simulink model "axi_qpsk_rx_tsync"  (R2017b)
settings: Solver=VariableStepAuto  StartTime=0.0  StopTime=10.0  RelTol=1e-3
PreLoadFcn:
  | fs_in = 25.6e6;
  | 
  | design_filters_rx;      % run script to generate filter designs.
  | 
  | Rb = 1000;   % 1kbit / s
  | 
  | Rsym = Rb/2;   % 2 bits per symbol
  | 
  | Rsymbol = Rb/2;
  | 
  | OSR = 32;
  | 
  | f_error = 120;
  | 
  | fc = 100e3;
undefined symbols (not defined in the file or in its folder): AXI4, Lite
libraries: xbsIndex_r4 x239
(part 1 of 2)
settings Model: Creator=jgoldsmi  LastModifiedBy=jgoldsmi

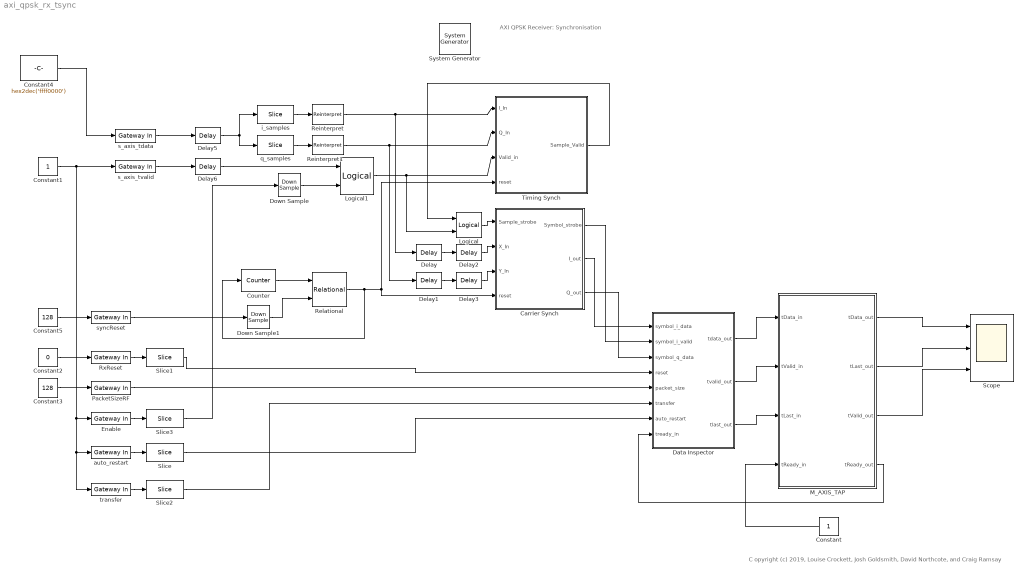
== system axi_qpsk_rx_tsync ==
  note: C opyright (c) 2019, Louise Crockett, Josh Goldsmith, David Northcote, and Craig Ramsay
  note: AXI QPSK Receiver:
      | Synchronisation
  " System Generator" : xbsIndex_r4/ System Generator  Tag=genX  xilinxfamily=zynquplusRFSOC  part=xczu28dr  speed=-2-e  package=ffvg1517  synthesis_tool=Vivado  clock_wrapper=Clock Enables  directory=Y:/git/craig_repo/rfsoc_qpsk_demo/boards/ip/sysgen/iprepo/zcu111/rx_stages/rx_tsync  proj_type=Vivado  Synth_file=Vivado Synthesis Defaults  Impl_file=Vivado Implementation Defaults  testbench=off  simulink_period=1/fs_in  sysclk_period=(1/fs_in)/1e-9  dcm_input_clock_period=10  incr_netlist=off  trim_vbits=Everywhere in SubSystem  dbl_ovrd=According to Block Masks  core_generation=According to Block Masks  run_coregen=off  deprecated_control=off  eval_field=0  block_type=sysgen
  Carrier Synch : Subsystem  mask(Symbol Timing Synchroniser){Rsymbol=Rsymbol}
      mask prompts: Rsymbol "Symbol rate (Hz)"
      mask init:
      | d = 0.707;                  % damping ratio 
      | 
      | % *** CARRIER synch loop *** (note this operates at symbol rate)
      | 
      | T = 1/Rsymbol;               % sample period
      | Kp = 1;                      % phase detector S-curve is linear
      | Bn = 0.04*Rsymbol;           % bandwidth in Hz
      | Ko = 1;                      % gain of NCO 
      | 
      | % calculate the loop filter coefficients for the carrier synch loop
      | K1 = (4*d*Bn*T)/(Ko*Kp*(d+1/(4*d)));
      | K2 = (4*(Bn*T)^2)/(Ko*Kp*(d+1/4*d)^2);
  Constant : Constant  OutDataTypeStr=boolean  SampleTime=1/fs_in
  Constant1 : Constant  OutDataTypeStr=boolean  SampleTime=-1
  Constant2 : Constant  Value=0  OutDataTypeStr=boolean  SampleTime=-1
  Constant3 : Constant  Value=128  OutDataTypeStr=uint32  SampleTime=-1
  Constant4 : Constant  Value=hex2dec('ffff0000')  OutDataTypeStr=uint32  SampleTime=1/fs_in
  Constant5 : Constant  Value=128  OutDataTypeStr=uint32  SampleTime=-1
  Counter : xbsIndex_r4/Counter  cnt_type=Free Running  cnt_to=Inf  operation=Up  start_count=1  cnt_by_val=1  arith_type=Unsigned  n_bits=32  bin_pt=0  load_pin=off  rst=on  en=off  explicit_period=on  period=1/16e3  use_behavioral_HDL=off  implementation=Fabric  dbl_ovrd=off  block_type=counter
  Data Inspector : Subsystem
  Delay : xbsIndex_r4/Delay  rst=off  infoeditControl=Selection of Reset will increase slice count due to use of real FFs and instead of SRLs  en=off  latency=OSR/2  reg_retiming=off  dbl_ovrd=off  block_type=delay
  Delay1 : xbsIndex_r4/Delay  rst=off  infoeditControl=Selection of Reset will increase slice count due to use of real FFs and instead of SRLs  en=off  latency=OSR/2  reg_retiming=off  dbl_ovrd=off  block_type=delay
  Delay{2..3,5..6} (4 alike) : xbsIndex_r4/Delay  rst=off  infoeditControl=Selection of Reset will increase slice count due to use of real FFs and instead of SRLs  en=off  latency=1  reg_retiming=off  dbl_ovrd=off  block_type=delay
  Down Sample : xbsIndex_r4/Down Sample  sample_ratio=1600  sample_phase="Last Value of Frame  (most efficient)"  en=off  rst=off  latency=1  dbl_ovrd=off  block_type=dsamp
  Down Sample1 : xbsIndex_r4/Down Sample  sample_ratio=1600  sample_phase="Last Value of Frame  (most efficient)"  en=off  rst=off  latency=1  dbl_ovrd=off  block_type=dsamp
  Enable : xbsIndex_r4/Gateway In  gui_display_data_type=Fixed-point  arith_type=Unsigned  n_bits=32  bin_pt=0  preci_type=Single  exp_width=8  frac_width=24  rows=1  columns=1  quantization="Round  (unbiased: +/- Inf)"  overflow=Saturate  period=1/fs_in  UseAsADC=off  ADCChannel='1'  interface=AXI4-Lite  automatic_assignment=off  address_offset=8  intf_name=''  intf_description=''  default_value=0  timing_constraint=None  locs_specified=off  LOCs={}  io_standard={}  inherit_from_input=off  hdl_port=on  dbl_ovrd=off  block_type=gatewayin
  Logical : xbsIndex_r4/Logical  logical_function=AND  inputs=2  en=off  latency=0  precision=Full  arith_type=Unsigned  n_bits=16  bin_pt=0  align_bp=on  dbl_ovrd=off  block_type=logical
  Logical1 : xbsIndex_r4/Logical  logical_function=AND  inputs=2  en=off  latency=0  precision=Full  arith_type=Unsigned  n_bits=16  bin_pt=0  align_bp=on  dbl_ovrd=off  block_type=logical
  M_AXIS_TAP : Subsystem
  PacketSizeRF : xbsIndex_r4/Gateway In  gui_display_data_type=Fixed-point  arith_type=Unsigned  n_bits=32  bin_pt=0  preci_type=Single  exp_width=8  frac_width=24  rows=1  columns=1  quantization=Truncate  overflow=Wrap  period=1/fs_in  UseAsADC=off  ADCChannel='1'  interface=AXI4-Lite  automatic_assignment=off  address_offset=4  intf_name=''  intf_description=''  default_value=0  timing_constraint=None  locs_specified=off  LOCs={}  io_standard={}  inherit_from_input=off  hdl_port=on  dbl_ovrd=off  block_type=gatewayin
  Reinterpret : xbsIndex_r4/Reinterpret  force_arith_type=on  arith_type="Signed  (2's comp)"  force_bin_pt=on  bin_pt=14  block_type=reinterpret
  Reinterpret1 : xbsIndex_r4/Reinterpret  force_arith_type=on  arith_type="Signed  (2's comp)"  force_bin_pt=on  bin_pt=14  block_type=reinterpret
  Relational : xbsIndex_r4/Relational  mode=a=b  op_type=Bool  en=off  latency=0  dbl_ovrd=off  block_type=relational
  RxReset : xbsIndex_r4/Gateway In  gui_display_data_type=Fixed-point  arith_type=Unsigned  n_bits=32  bin_pt=0  preci_type=Single  exp_width=8  frac_width=24  rows=1  columns=1  quantization="Round  (unbiased: +/- Inf)"  overflow=Saturate  period=1/fs_in  UseAsADC=off  ADCChannel='1'  interface=AXI4-Lite  automatic_assignment=off  address_offset=0  intf_name=''  intf_description=''  default_value=0  timing_constraint=None  locs_specified=off  LOCs={}  io_standard={}  inherit_from_input=off  hdl_port=on  dbl_ovrd=off  block_type=gatewayin
  Scope : Scope  NumInputPorts=3
  Slice{,1..3} (4 alike) : xbsIndex_r4/Slice  nbits=1  boolean_output=on  mode=Two Bit Locations  bit1=0  base1=LSB of Input  bit0=0  base0=LSB of Input  dbl_ovrd=off  block_type=slice
  Timing Synch : Subsystem  mask(Symbol Timing Synchroniser){Rsymbol=Rsymbol}
      mask prompts: Rsymbol "Symbol rate (Hz)"
      mask init:
      | % *** SYMBOL TIMING synch loop ***
      | 
      | d = 0.707;                  % damping ratio 
      | Ts = 1/Rsymbol;             % symbol period
      | Ks = 3.24;                  % phase detector coefficient
      | BnS = 0.08*Rsymbol;         % bandwidth in Hz
      | Kn   = 1;                   % gain of numerically controlled clock
      | 
      | % calculate loop filter coefficients
      | Ka = (4*d*BnS*Ts)/(Kn*Ks*(d+1/(4*d)));
      | Kb = (4*(BnS*Ts)^2)/(Kn*Ks*(d+1/4*d)^2);
  auto_restart : xbsIndex_r4/Gateway In  gui_display_data_type=Fixed-point  arith_type=Unsigned  n_bits=32  bin_pt=0  preci_type=Single  exp_width=8  frac_width=24  rows=1  columns=1  quantization="Round  (unbiased: +/- Inf)"  overflow=Saturate  period=1/fs_in  UseAsADC=off  ADCChannel='1'  interface=AXI4-Lite  automatic_assignment=off  address_offset=12  intf_name=''  intf_description=''  default_value=0  timing_constraint=None  locs_specified=off  LOCs={}  io_standard={}  inherit_from_input=off  hdl_port=on  dbl_ovrd=off  block_type=gatewayin
  i_samples : xbsIndex_r4/Slice  nbits=16  boolean_output=off  mode=Upper Bit Location + Width  bit1=0  base1=MSB of Input  bit0=0  base0=LSB of Input  dbl_ovrd=off  block_type=slice
  q_samples : xbsIndex_r4/Slice  nbits=16  boolean_output=off  mode=Lower Bit Location + Width  bit1=0  base1=MSB of Input  bit0=0  base0=LSB of Input  dbl_ovrd=off  block_type=slice
  s_axis_tdata : xbsIndex_r4/Gateway In  gui_display_data_type=Fixed-point  arith_type=Unsigned  n_bits=32  bin_pt=0  preci_type=Single  exp_width=8  frac_width=24  rows=1  columns=1  quantization="Round  (unbiased: +/- Inf)"  overflow=Saturate  period=1/16e3  UseAsADC=off  ADCChannel='1'  interface=None  automatic_assignment=on  address_offset=hex2dec('00')  intf_name=''  intf_description=''  default_value=0  timing_constraint=None  locs_specified=off  LOCs={}  io_standard={}  inherit_from_input=off  hdl_port=on  dbl_ovrd=off  block_type=gatewayin
  s_axis_tvalid : xbsIndex_r4/Gateway In  gui_display_data_type=Boolean  arith_type=Boolean  n_bits=32  bin_pt=0  preci_type=Single  exp_width=8  frac_width=24  rows=1  columns=1  quantization="Round  (unbiased: +/- Inf)"  overflow=Saturate  period=1/16e3  UseAsADC=off  ADCChannel='1'  interface=None  automatic_assignment=on  address_offset=hex2dec('00')  intf_name=''  intf_description=''  default_value=0  timing_constraint=None  locs_specified=off  LOCs={}  io_standard={}  inherit_from_input=off  hdl_port=on  dbl_ovrd=off  block_type=gatewayin
  syncReset : xbsIndex_r4/Gateway In  gui_display_data_type=Fixed-point  arith_type=Unsigned  n_bits=32  bin_pt=0  preci_type=Single  exp_width=8  frac_width=24  rows=1  columns=1  quantization=Truncate  overflow=Wrap  period=1/fs_in  UseAsADC=off  ADCChannel='1'  interface=AXI4-Lite  automatic_assignment=off  address_offset=20  intf_name=''  intf_description=''  default_value=0  timing_constraint=None  locs_specified=off  LOCs={}  io_standard={}  inherit_from_input=off  hdl_port=on  dbl_ovrd=off  block_type=gatewayin
  transfer : xbsIndex_r4/Gateway In  gui_display_data_type=Fixed-point  arith_type=Unsigned  n_bits=32  bin_pt=0  preci_type=Single  exp_width=8  frac_width=24  rows=1  columns=1  quantization="Round  (unbiased: +/- Inf)"  overflow=Saturate  period=1/fs_in  UseAsADC=off  ADCChannel='1'  interface=AXI4-Lite  automatic_assignment=off  address_offset=16  intf_name=''  intf_description=''  default_value=0  timing_constraint=None  locs_specified=off  LOCs={}  io_standard={}  inherit_from_input=off  hdl_port=on  dbl_ovrd=off  block_type=gatewayin
  wires:
  RxReset/1 -> Slice1/1
  Enable/1 -> Slice3/1
  auto_restart/1 -> Slice/1
  transfer/1 -> Slice2/1
  Constant2/1 -> RxReset/1
  Constant1/1 -> transfer/1, auto_restart/1, Enable/1, s_axis_tvalid/1
  Constant3/1 -> PacketSizeRF/1
  M_AXIS_TAP/3(tValid_out) -> Scope/3
  Constant/1 -> M_AXIS_TAP/4(tReady_in)
  Data Inspector/3(tlast_out) -> M_AXIS_TAP/3(tLast_in)
  M_AXIS_TAP/1(tData_out) -> Scope/1
  M_AXIS_TAP/2(tLast_out) -> Scope/2
  M_AXIS_TAP/4(tReady_out) -> Data Inspector/8(tready_in)
  Data Inspector/2(tvalid_out) -> M_AXIS_TAP/2(tValid_in)
  Data Inspector/1(tdata_out) -> M_AXIS_TAP/1(tData_in)
  Delay/1 -> Delay2/1
  Delay3/1 -> Carrier Synch/3(Y_In)
  Delay2/1 -> Carrier Synch/2(X_In)
  Timing Synch/1(Sample_Valid) -> Logical/1
  Logical/1 -> Carrier Synch/1(Sample_strobe)
  Delay1/1 -> Delay3/1
  i_samples/1 -> Reinterpret/1
  q_samples/1 -> Reinterpret1/1
  Slice1/1 -> Data Inspector/4(reset)
  PacketSizeRF/1 -> Data Inspector/5(packet_size)
  Logical1/1 -> Logical/2, Timing Synch/3(Valid_in)
  Slice3/1 -> Down Sample/1
  Slice/1 -> Data Inspector/7(auto_restart)
  Slice2/1 -> Data Inspector/6(transfer)
  Carrier Synch/1(Symbol_strobe) -> Data Inspector/2(symbol_i_valid)
  Down Sample/1 -> Logical1/2
  Constant4/1 -> s_axis_tdata/1
  Carrier Synch/2(I_out) -> Data Inspector/1(symbol_i_data)
  Carrier Synch/3(Q_out) -> Data Inspector/3(symbol_q_data)
  Constant5/1 -> syncReset/1
  s_axis_tdata/1 -> Delay5/1
  s_axis_tvalid/1 -> Delay6/1
  Reinterpret/1 -> Delay/1, Timing Synch/1(I_In)
  Reinterpret1/1 -> Delay1/1, Timing Synch/2(Q_In)
  Delay6/1 -> Logical1/1
  Delay5/1 -> q_samples/1, i_samples/1
  syncReset/1 -> Down Sample1/1
  Relational/1 -> Counter/1, Carrier Synch/4(reset), Timing Synch/4(reset)
  Counter/1 -> Relational/1
  Down Sample1/1 -> Relational/2

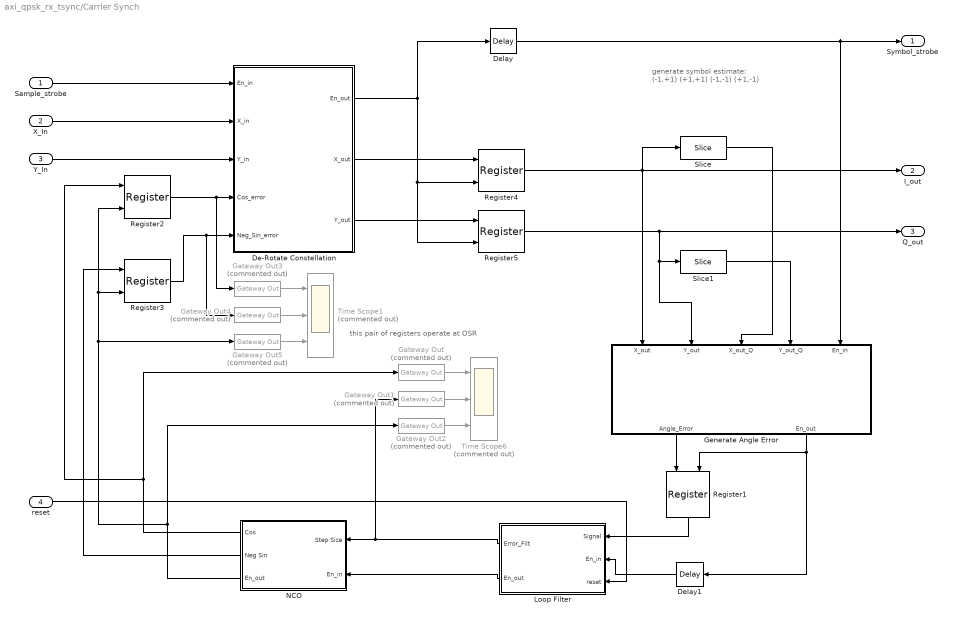
== system axi_qpsk_rx_tsync/Carrier Synch ==
  note: this pair of registers operate at OSR
  note: generate symbol estimate:
      |
      |           (-1,+1)                 (+1,+1)
      |
      |
      |           (-1,-1)                  (+1,-1)
  Sample_strobe : Inport
  X_In : Inport  Port=2
  Y_In : Inport  Port=3
  reset : Inport  Port=4
  De-Rotate Constellation : Subsystem
  Delay : xbsIndex_r4/Delay  rst=off  infoeditControl=Selection of Reset will increase slice count due to use of real FFs and instead of SRLs  en=off  latency=1  reg_retiming=off  dbl_ovrd=off  block_type=delay
  Delay1 : xbsIndex_r4/Delay  rst=off  infoeditControl=Selection of Reset will increase slice count due to use of real FFs and instead of SRLs  en=off  latency=1  reg_retiming=off  dbl_ovrd=off  block_type=delay
  Gateway Out{,1..5} (6 alike) : xbsIndex_r4/Gateway Out  Commented=on  inherit_from_input=off  hdl_port=on  rows=1  columns=1  UseAsDAC=off  DACChannel='1'  interface=None  automatic_assignment=on  address_offset=hex2dec('00')  intf_name=''  intf_description=''  timing_constraint=None  locs_specified=off  LOCs={}  io_standard={}  block_type=gatewayout
  Generate Angle Error : Subsystem
  Loop Filter : Subsystem  mask(Loop Filter){K1=K1, K2=K2}
      mask prompts: K1 "Proportional gain (K1)"; K2 "Integral gain (K2)"
      mask help:
      | Filters the error signal generated within the Carrier Synchronisation Loop.
      |
      | Key parameters are the gain of the proportional and integral branches.
  NCO : Subsystem  mask(NCO){n=8, b=14}
      mask prompts: n "Number of integer_bits"; b "Number of fractional bits"
      mask help:
      | Numerically Controller Oscillator.
      |
      | Integrates the phase error and generates cosine and negative sign outputs.
      mask init:
      | k_n = ceil(log2((2^n)/(2*pi)))
      mask DialogControl Container3 Prompt: Accumulator
  Register1 : xbsIndex_r4/Register  init=0  rst=off  en=on  dbl_ovrd=off  block_type=register
  Register2 : xbsIndex_r4/Register  init=1  rst=off  en=on  dbl_ovrd=off  block_type=register
  Register3 : xbsIndex_r4/Register  init=0  rst=off  en=on  dbl_ovrd=off  block_type=register
  Register4 : xbsIndex_r4/Register  init=1  rst=off  en=on  dbl_ovrd=off  block_type=register
  Register5 : xbsIndex_r4/Register  init=1  rst=off  en=on  dbl_ovrd=off  block_type=register
  Slice : xbsIndex_r4/Slice  nbits=1  boolean_output=off  mode=Upper Bit Location + Width  bit1=0  base1=MSB of Input  bit0=0  base0=LSB of Input  dbl_ovrd=off  block_type=slice
  Slice1 : xbsIndex_r4/Slice  nbits=1  boolean_output=off  mode=Upper Bit Location + Width  bit1=0  base1=MSB of Input  bit0=0  base0=LSB of Input  dbl_ovrd=off  block_type=slice
  Time Scope1 : Scope  Commented=on  NumInputPorts=3
  Time Scope6 : Scope  Commented=on  NumInputPorts=3
  Symbol_strobe : Outport
  I_out : Outport  Port=2
  Q_out : Outport  Port=3
  wires:
  X_In/1 -> De-Rotate Constellation/2(X_in)
  Y_In/1 -> De-Rotate Constellation/3(Y_in)
  Register4/1 -> Slice/1, I_out/1, Generate Angle Error/1(X_out)
  Register5/1 -> Q_out/1, Generate Angle Error/2(Y_out), Slice1/1
  Slice/1 -> Generate Angle Error/3(X_out_Q)
  Slice1/1 -> Generate Angle Error/4(Y_out_Q)
  Register1/1 -> Loop Filter/1(Signal)
  Loop Filter/2(En_out) -> NCO/2(En_in)
  Loop Filter/1(Error_Filt) -> Gateway Out1/1, NCO/1(Step Size)
  Register2/1 -> Gateway Out3/1, De-Rotate Constellation/4(Cos_error)
  Register3/1 -> Gateway Out4/1, De-Rotate Constellation/5(Neg_Sin_error)
  NCO/1(Cos) -> Gateway Out/1, Register2/1
  NCO/2(Neg Sin) -> Register3/1
  NCO/3(En_out) -> Gateway Out2/1, Gateway Out5/1, Register2/2, Register3/2
  Sample_strobe/1 -> De-Rotate Constellation/1(En_in)
  De-Rotate Constellation/1(En_out) -> Delay/1, Register4/2, Register5/2
  Delay/1 -> Symbol_strobe/1, Generate Angle Error/5(En_in)
  Gateway Out/1 -> Time Scope6/1
  Gateway Out1/1 -> Time Scope6/2
  Gateway Out2/1 -> Time Scope6/3
  Generate Angle Error/1(Angle_Error) -> Register1/1
  Generate Angle Error/2(En_out) -> Delay1/1, Register1/2
  Delay1/1 -> Loop Filter/2(En_in)
  Gateway Out5/1 -> Time Scope1/3
  Gateway Out4/1 -> Time Scope1/2
  Gateway Out3/1 -> Time Scope1/1
  De-Rotate Constellation/2(X_out) -> Register4/1
  De-Rotate Constellation/3(Y_out) -> Register5/1
  reset/1 -> Loop Filter/3(reset)

== system axi_qpsk_rx_tsync/Data Inspector ==
  symbol_i_data : Inport
  symbol_i_valid : Inport  Port=2
  symbol_q_data : Inport  Port=3
  reset : Inport  Port=4
  packet_size : Inport  Port=5
  transfer : Inport  Port=6
  auto_restart : Inport  Port=7
  tready_in : Inport  Port=8
  M_AXIS_SYMBOL_CTRL : Subsystem
  tdata_out : Outport
  tvalid_out : Outport  Port=2
  tlast_out : Outport  Port=3
  wires:
  auto_restart/1 -> M_AXIS_SYMBOL_CTRL/8(auto_restart)
  transfer/1 -> M_AXIS_SYMBOL_CTRL/7(transfer)
  M_AXIS_SYMBOL_CTRL/3(tlast_out) -> tlast_out/1
  M_AXIS_SYMBOL_CTRL/2(tvalid_out) -> tvalid_out/1
  M_AXIS_SYMBOL_CTRL/1(tdata_out) -> tdata_out/1
  tready_in/1 -> M_AXIS_SYMBOL_CTRL/6(tready_in)
  packet_size/1 -> M_AXIS_SYMBOL_CTRL/5(packet_size)
  reset/1 -> M_AXIS_SYMBOL_CTRL/4(reset)
  symbol_q_data/1 -> M_AXIS_SYMBOL_CTRL/3(q_data)
  symbol_i_valid/1 -> M_AXIS_SYMBOL_CTRL/2(tvalid_in)
  symbol_i_data/1 -> M_AXIS_SYMBOL_CTRL/1(i_data)

== system axi_qpsk_rx_tsync/M_AXIS_TAP ==
  tData_in : Inport
  tValid_in : Inport  Port=2
  tLast_in : Inport  Port=3
  tReady_in : Inport  Port=4
  m_axis_tap_tdata : xbsIndex_r4/Gateway Out  inherit_from_input=off  hdl_port=on  rows=1  columns=1  UseAsDAC=off  DACChannel='1'  interface=None  automatic_assignment=on  address_offset=hex2dec('00')  intf_name=''  intf_description=''  timing_constraint=None  locs_specified=off  LOCs={}  io_standard={}  block_type=gatewayout
  m_axis_tap_tlast : xbsIndex_r4/Gateway Out  inherit_from_input=off  hdl_port=on  rows=1  columns=1  UseAsDAC=off  DACChannel='1'  interface=None  automatic_assignment=on  address_offset=hex2dec('00')  intf_name=''  intf_description=''  timing_constraint=None  locs_specified=off  LOCs={}  io_standard={}  block_type=gatewayout
  m_axis_tap_tready : xbsIndex_r4/Gateway In  gui_display_data_type=Boolean  arith_type=Boolean  n_bits=16  bin_pt=14  preci_type=Single  exp_width=8  frac_width=24  rows=1  columns=1  quantization="Round  (unbiased: +/- Inf)"  overflow=Saturate  period=1/fs_in  UseAsADC=off  ADCChannel='1'  interface=None  automatic_assignment=on  address_offset=hex2dec('00')  intf_name=''  intf_description=''  default_value=0  timing_constraint=None  locs_specified=off  LOCs={}  io_standard={}  inherit_from_input=off  hdl_port=on  dbl_ovrd=off  block_type=gatewayin
  m_axis_tap_tvalid : xbsIndex_r4/Gateway Out  inherit_from_input=off  hdl_port=on  rows=1  columns=1  UseAsDAC=off  DACChannel='1'  interface=None  automatic_assignment=on  address_offset=hex2dec('00')  intf_name=''  intf_description=''  timing_constraint=None  locs_specified=off  LOCs={}  io_standard={}  block_type=gatewayout
  tData_out : Outport
  tLast_out : Outport  Port=2
  tValid_out : Outport  Port=3
  tReady_out : Outport  Port=4
  wires:
  m_axis_tap_tready/1 -> tReady_out/1
  tValid_in/1 -> m_axis_tap_tvalid/1
  tLast_in/1 -> m_axis_tap_tlast/1
  tData_in/1 -> m_axis_tap_tdata/1
  m_axis_tap_tdata/1 -> tData_out/1
  m_axis_tap_tvalid/1 -> tValid_out/1
  m_axis_tap_tlast/1 -> tLast_out/1
  tReady_in/1 -> m_axis_tap_tready/1

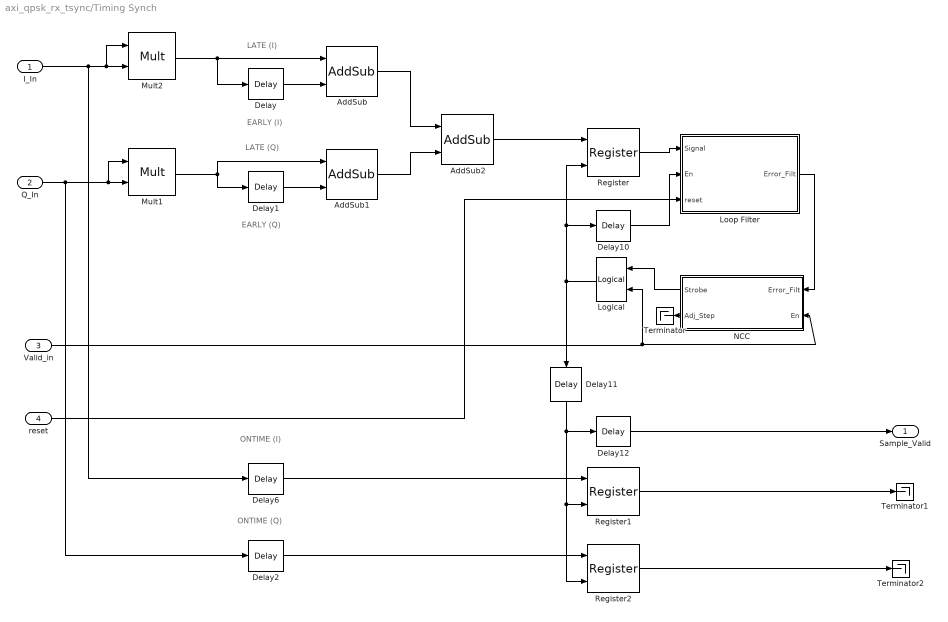
== system axi_qpsk_rx_tsync/Timing Synch ==
  note: LATE (I)
  note: LATE (Q)
  note: EARLY (I)
  note: EARLY (Q)
  note: ONTIME (I)
  note: ONTIME (Q)
  I_In : Inport
  Q_In : Inport  Port=2
  Valid_in : Inport  Port=3
  reset : Inport  Port=4
  AddSub : xbsIndex_r4/AddSub  mode=Subtraction  use_carryin=off  use_carryout=off  en=off  latency=0  precision=Full  arith_type=Unsigned  n_bits=16  bin_pt=14  quantization=Truncate  overflow=Wrap  use_behavioral_HDL=off  hw_selection=Fabric  pipelined=off  dbl_ovrd=off  block_type=addsub
  AddSub1 : xbsIndex_r4/AddSub  mode=Subtraction  use_carryin=off  use_carryout=off  en=off  latency=0  precision=Full  arith_type=Unsigned  n_bits=16  bin_pt=14  quantization=Truncate  overflow=Wrap  use_behavioral_HDL=off  hw_selection=Fabric  pipelined=off  dbl_ovrd=off  block_type=addsub
  AddSub2 : xbsIndex_r4/AddSub  mode=Addition  use_carryin=off  use_carryout=off  en=off  latency=0  precision=Full  arith_type=Unsigned  n_bits=16  bin_pt=14  quantization=Truncate  overflow=Wrap  use_behavioral_HDL=off  hw_selection=Fabric  pipelined=off  dbl_ovrd=off  block_type=addsub
  Delay : xbsIndex_r4/Delay  rst=off  infoeditControl=Selection of Reset will increase slice count due to use of real FFs and instead of SRLs  en=off  latency=OSR  reg_retiming=off  dbl_ovrd=off  block_type=delay
  Delay1 : xbsIndex_r4/Delay  rst=off  infoeditControl=Selection of Reset will increase slice count due to use of real FFs and instead of SRLs  en=off  latency=OSR  reg_retiming=off  dbl_ovrd=off  block_type=delay
  Delay10 : xbsIndex_r4/Delay  rst=off  infoeditControl=Selection of Reset will increase slice count due to use of real FFs and instead of SRLs  en=off  latency=1  reg_retiming=off  dbl_ovrd=off  block_type=delay
  Delay11 : xbsIndex_r4/Delay  rst=off  infoeditControl=Selection of Reset will increase slice count due to use of real FFs and instead of SRLs  en=off  latency=OSR/2  reg_retiming=off  dbl_ovrd=off  block_type=delay
  Delay12 : xbsIndex_r4/Delay  rst=off  infoeditControl=Selection of Reset will increase slice count due to use of real FFs and instead of SRLs  en=off  latency=1  reg_retiming=off  dbl_ovrd=off  block_type=delay
  Delay2 : xbsIndex_r4/Delay  rst=off  infoeditControl=Selection of Reset will increase slice count due to use of real FFs and instead of SRLs  en=off  latency=OSR/2  reg_retiming=off  dbl_ovrd=off  block_type=delay
  Delay6 : xbsIndex_r4/Delay  rst=off  infoeditControl=Selection of Reset will increase slice count due to use of real FFs and instead of SRLs  en=off  latency=OSR/2  reg_retiming=off  dbl_ovrd=off  block_type=delay
  Logical : xbsIndex_r4/Logical  logical_function=AND  inputs=2  en=off  latency=0  precision=Full  arith_type=Unsigned  n_bits=16  bin_pt=0  align_bp=on  dbl_ovrd=off  block_type=logical
  Loop Filter : Subsystem  mask(Loop Filter){Ka=Ka, Kb=Kb}
      mask prompts: Ka "Proportional gain (Ka)"; Kb "Integral gain (Kb)"
      mask help:
      | Filters the error signal generated by the Timing Error Detector.
      |
      | Key parameters are the gain of the proportional and integral branches.
  Mult1 : xbsIndex_r4/Mult  precision=User Defined  arith_type="Signed  (2's comp)"  n_bits=18  bin_pt=14  quantization=Truncate  overflow=Wrap  en=off  latency=0  use_behavioral_HDL=off  opt=Speed  use_embedded=on  optimum_pipeline=off  pipeline=on  dbl_ovrd=off  use_rpm=on  placement_style=Triangular  block_type=mult
  Mult2 : xbsIndex_r4/Mult  precision=User Defined  arith_type="Signed  (2's comp)"  n_bits=18  bin_pt=14  quantization=Truncate  overflow=Wrap  en=off  latency=0  use_behavioral_HDL=off  opt=Speed  use_embedded=on  optimum_pipeline=off  pipeline=on  dbl_ovrd=off  use_rpm=on  placement_style=Triangular  block_type=mult
  NCC : Subsystem  mask(Numerically Controlled Clock (NCC)){OSR=OSR, b=24}
      mask prompts: OSR "Oversampling ratio (nominal samples per symbol)"; b "Fractional bits"
      mask help: Creates strobes at a rate matching the symbol rate of the received data.
      mask init:
      | n = ceil(log2(OSR));
  Register : xbsIndex_r4/Register  init=0  rst=off  en=on  dbl_ovrd=off  block_type=register
  Register1 : xbsIndex_r4/Register  init=0  rst=off  en=on  dbl_ovrd=off  block_type=register
  Register2 : xbsIndex_r4/Register  init=0  rst=off  en=on  dbl_ovrd=off  block_type=register
  Terminator : Terminator
  Terminator1 : Terminator
  Terminator2 : Terminator
  Sample_Valid : Outport
  wires:
  Delay11/1 -> Register2/2, Register1/2, Delay12/1
  Delay/1 -> AddSub/2
  AddSub1/1 -> AddSub2/2
  Mult2/1 -> AddSub/1, Delay/1
  AddSub2/1 -> Register/1
  I_In/1 -> Delay6/1, Mult2/2, Mult2/1
  Q_In/1 -> Delay2/1, Mult1/1, Mult1/2
  Delay10/1 -> Loop Filter/2(En)
  Loop Filter/1(Error_Filt) -> NCC/1(Error_Filt)
  Delay2/1 -> Register2/1
  Delay6/1 -> Register1/1
  Mult1/1 -> Delay1/1, AddSub1/1
  AddSub/1 -> AddSub2/1
  Delay1/1 -> AddSub1/2
  Logical/1 -> Delay11/1, Register/2, Delay10/1
  Register/1 -> Loop Filter/1(Signal)
  Register2/1 -> Terminator2/1
  Delay12/1 -> Sample_Valid/1
  NCC/1(Strobe) -> Logical/1
  Valid_in/1 -> NCC/2(En), Logical/2
  NCC/2(Adj_Step) -> Terminator/1
  Register1/1 -> Terminator1/1
  reset/1 -> Loop Filter/3(reset)

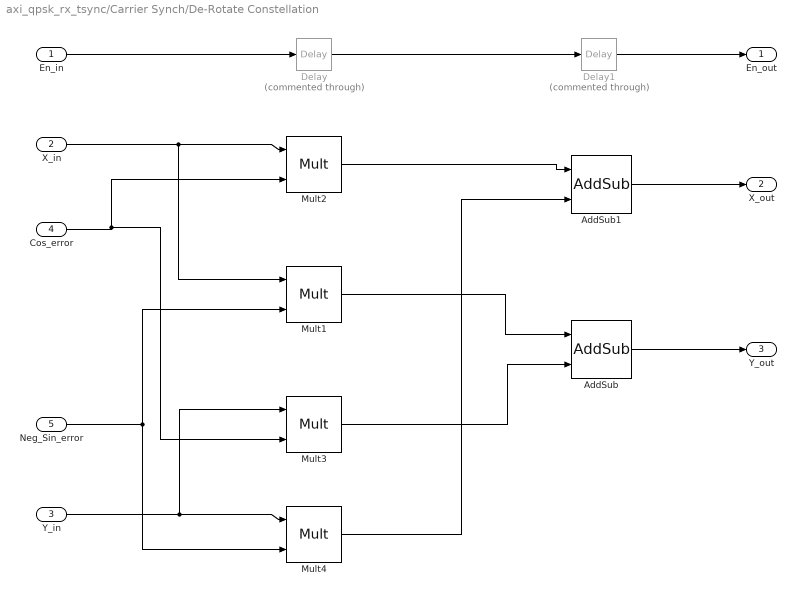
== system axi_qpsk_rx_tsync/Carrier Synch/De-Rotate Constellation ==
  En_in : Inport
  X_in : Inport  Port=2
  Y_in : Inport  Port=3
  Cos_error : Inport  Port=4
  Neg_Sin_error : Inport  Port=5
  AddSub : xbsIndex_r4/AddSub  mode=Addition  use_carryin=off  use_carryout=off  en=off  latency=0  precision=Full  arith_type=Unsigned  n_bits=16  bin_pt=14  quantization=Truncate  overflow=Wrap  use_behavioral_HDL=off  hw_selection=Fabric  pipelined=off  dbl_ovrd=off  block_type=addsub
  AddSub1 : xbsIndex_r4/AddSub  mode=Subtraction  use_carryin=off  use_carryout=off  en=off  latency=0  precision=Full  arith_type=Unsigned  n_bits=16  bin_pt=14  quantization=Truncate  overflow=Wrap  use_behavioral_HDL=off  hw_selection=Fabric  pipelined=off  dbl_ovrd=off  block_type=addsub
  Delay : xbsIndex_r4/Delay  Commented=through  rst=off  infoeditControl=Selection of Reset will increase slice count due to use of real FFs and instead of SRLs  en=off  latency=1  reg_retiming=off  dbl_ovrd=off  block_type=delay
  Delay1 : xbsIndex_r4/Delay  Commented=through  rst=off  infoeditControl=Selection of Reset will increase slice count due to use of real FFs and instead of SRLs  en=off  latency=1  reg_retiming=off  dbl_ovrd=off  block_type=delay
  Mult{1..4} (4 alike) : xbsIndex_r4/Mult  precision=User Defined  arith_type="Signed  (2's comp)"  n_bits=18  bin_pt=14  quantization=Truncate  overflow=Wrap  en=off  latency=0  use_behavioral_HDL=off  opt=Speed  use_embedded=on  optimum_pipeline=off  pipeline=on  dbl_ovrd=off  use_rpm=on  placement_style=Triangular  block_type=mult
  En_out : Outport
  X_out : Outport  Port=2
  Y_out : Outport  Port=3
  wires:
  AddSub1/1 -> X_out/1
  Y_in/1 -> Mult3/1, Mult4/1
  Mult2/1 -> AddSub1/1
  Mult3/1 -> AddSub/2
  Cos_error/1 -> Mult3/2, Mult2/2
  X_in/1 -> Mult1/1, Mult2/1
  Mult1/1 -> AddSub/1
  AddSub/1 -> Y_out/1
  Mult4/1 -> AddSub1/2
  Neg_Sin_error/1 -> Mult4/2, Mult1/2
  En_in/1 -> Delay/1
  Delay/1 -> Delay1/1
  Delay1/1 -> En_out/1

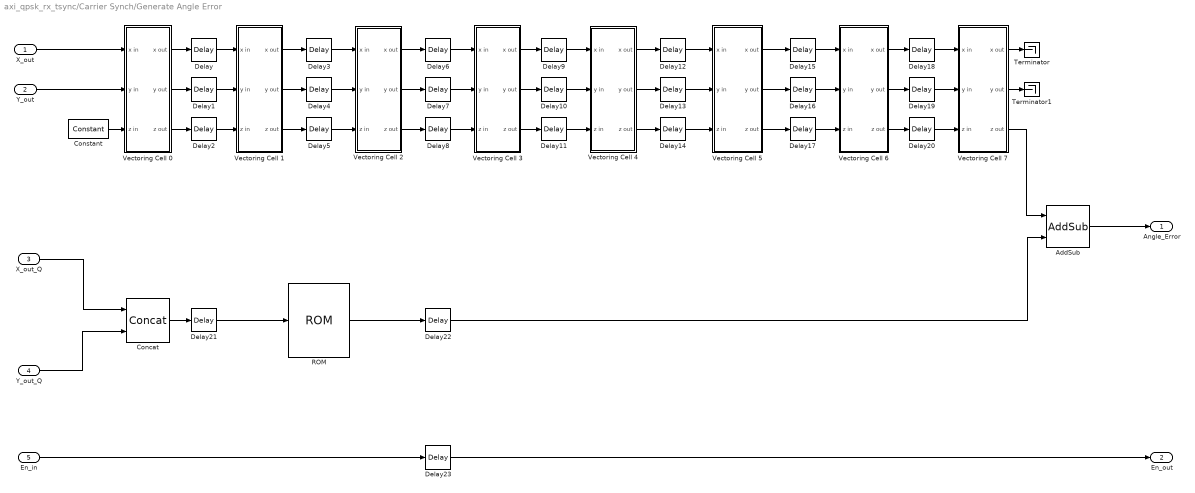
== system axi_qpsk_rx_tsync/Carrier Synch/Generate Angle Error ==
  X_out : Inport
  Y_out : Inport  Port=2
  X_out_Q : Inport  Port=3
  Y_out_Q : Inport  Port=4
  En_in : Inport  Port=5
  AddSub : xbsIndex_r4/AddSub  mode=Subtraction  use_carryin=off  use_carryout=off  en=off  latency=1  precision=Full  arith_type=Unsigned  n_bits=16  bin_pt=14  quantization=Truncate  overflow=Wrap  use_behavioral_HDL=off  hw_selection=Fabric  pipelined=off  dbl_ovrd=off  block_type=addsub
  Concat : xbsIndex_r4/Concat  num_inputs=2  dbl_ovrd=off  block_type=concat
  Constant : xbsIndex_r4/Constant  const=0  gui_display_data_type=Fixed-point  arith_type=Signed (2's comp)  n_bits=16  bin_pt=14  preci_type=Single  exp_width=8  frac_width=24  explicit_period=off  period=1  equ=P=C  opselect=C  inp2=PCIN>>17  opr=+  inp1=P  carry=CIN  dbl_ovrd=off  block_type=constant
  Delay{,1..21} (22 alike) : xbsIndex_r4/Delay  rst=off  infoeditControl=Selection of Reset will increase slice count due to use of real FFs and instead of SRLs  en=off  latency=1  reg_retiming=off  dbl_ovrd=off  block_type=delay
  Delay22 : xbsIndex_r4/Delay  rst=off  infoeditControl=Selection of Reset will increase slice count due to use of real FFs and instead of SRLs  en=off  latency=5  reg_retiming=off  dbl_ovrd=off  block_type=delay
  Delay23 : xbsIndex_r4/Delay  rst=off  infoeditControl=Selection of Reset will increase slice count due to use of real FFs and instead of SRLs  en=off  latency=8  reg_retiming=off  dbl_ovrd=off  block_type=delay
  ROM : xbsIndex_r4/ROM  depth=4  initVector=[pi/4 -pi/4 -pi/4 pi/4]  distributed_mem=Block RAM  rst=off  init_reg=0  en=off  latency=1  gui_display_data_type=Fixed-point  arith_type="Signed  (2's comp)"  n_bits=16  bin_pt=14  preci_type=Single  exp_width=8  frac_width=24  optimize=Area  use_rpm=on  dbl_ovrd=off  block_type=sprom
  Terminator : Terminator
  Terminator1 : Terminator
  Vectoring Cell 2 : Subsystem  mask(Cordic Vectoring Cell){i=2}
      mask prompts: i "Iteration Number (i)"
      mask help: some notes to go here
  Vectoring Cell 3 : Subsystem  mask(Cordic Vectoring Cell){i=3}
      mask prompts: i "Iteration Number (i)"
      mask help: some notes to go here
  Vectoring Cell 4 : Subsystem  mask(Cordic Vectoring Cell){i=4}
      mask prompts: i "Iteration Number (i)"
      mask help: some notes to go here
  Vectoring Cell 5 : Subsystem  mask(Cordic Vectoring Cell){i=5}
      mask prompts: i "Iteration Number (i)"
      mask help: some notes to go here
  Vectoring Cell 6 : Subsystem  mask(Cordic Vectoring Cell){i=6}
      mask prompts: i "Iteration Number (i)"
      mask help: some notes to go here
  Vectoring Cell 7 : Subsystem  mask(Cordic Vectoring Cell){i=7}
      mask prompts: i "Iteration Number (i)"
      mask help: some notes to go here
  Vectoring Cell 0 : Subsystem  mask(Cordic Vectoring Cell){i=0}
      mask prompts: i "Iteration Number (i)"
      mask help: some notes to go here
  Vectoring Cell 1 : Subsystem  mask(Cordic Vectoring Cell){i=1}
      mask prompts: i "Iteration Number (i)"
      mask help: some notes to go here
  Angle_Error : Outport
  En_out : Outport  Port=2
  wires:
  X_out_Q/1 -> Concat/1
  Y_out_Q/1 -> Concat/2
  Concat/1 -> Delay21/1
  Vectoring Cell 0/2(y out) -> Delay1/1
  Vectoring Cell 3/1(x out) -> Delay9/1
  Vectoring Cell 6/1(x out) -> Delay18/1
  Vectoring Cell 1/3(z out) -> Delay5/1
  Vectoring Cell 3/3(z out) -> Delay11/1
  Vectoring Cell 5/3(z out) -> Delay17/1
  Vectoring Cell 1/2(y out) -> Delay4/1
  Vectoring Cell 4/1(x out) -> Delay12/1
  Vectoring Cell 1/1(x out) -> Delay3/1
  X_out/1 -> Vectoring Cell 0/1(x in)
  Vectoring Cell 2/2(y out) -> Delay7/1
  Vectoring Cell 2/1(x out) -> Delay6/1
  Vectoring Cell 5/2(y out) -> Delay16/1
  Vectoring Cell 0/3(z out) -> Delay2/1
  Vectoring Cell 3/2(y out) -> Delay10/1
  Vectoring Cell 2/3(z out) -> Delay8/1
  Vectoring Cell 4/2(y out) -> Delay13/1
  Vectoring Cell 4/3(z out) -> Delay14/1
  Vectoring Cell 5/1(x out) -> Delay15/1
  Vectoring Cell 0/1(x out) -> Delay/1
  Constant/1 -> Vectoring Cell 0/3(z in)
  Delay/1 -> Vectoring Cell 1/1(x in)
  Delay1/1 -> Vectoring Cell 1/2(y in)
  Delay2/1 -> Vectoring Cell 1/3(z in)
  Delay3/1 -> Vectoring Cell 2/1(x in)
  Delay4/1 -> Vectoring Cell 2/2(y in)
  Delay5/1 -> Vectoring Cell 2/3(z in)
  Delay6/1 -> Vectoring Cell 3/1(x in)
  Delay7/1 -> Vectoring Cell 3/2(y in)
  Delay8/1 -> Vectoring Cell 3/3(z in)
  Delay9/1 -> Vectoring Cell 4/1(x in)
  Delay10/1 -> Vectoring Cell 4/2(y in)
  Delay11/1 -> Vectoring Cell 4/3(z in)
  Delay12/1 -> Vectoring Cell 5/1(x in)
  Delay13/1 -> Vectoring Cell 5/2(y in)
  Delay14/1 -> Vectoring Cell 5/3(z in)
  Delay15/1 -> Vectoring Cell 6/1(x in)
  Delay16/1 -> Vectoring Cell 6/2(y in)
  Delay17/1 -> Vectoring Cell 6/3(z in)
  Delay20/1 -> Vectoring Cell 7/3(z in)
  Delay19/1 -> Vectoring Cell 7/2(y in)
  Delay18/1 -> Vectoring Cell 7/1(x in)
  Vectoring Cell 6/2(y out) -> Delay19/1
  Vectoring Cell 6/3(z out) -> Delay20/1
  Vectoring Cell 7/2(y out) -> Terminator1/1
  Vectoring Cell 7/1(x out) -> Terminator/1
  Vectoring Cell 7/3(z out) -> AddSub/1
  ROM/1 -> Delay22/1
  AddSub/1 -> Angle_Error/1
  Delay21/1 -> ROM/1
  Delay22/1 -> AddSub/2
  En_in/1 -> Delay23/1
  Delay23/1 -> En_out/1
  Y_out/1 -> Vectoring Cell 0/2(y in)

== system axi_qpsk_rx_tsync/Carrier Synch/Loop Filter ==
  Signal : Inport
  En_in : Inport  Port=2
  reset : Inport  Port=3
  AddSub3 : xbsIndex_r4/AddSub  mode=Addition  use_carryin=off  use_carryout=off  en=off  latency=0  precision=User Defined  arith_type="Signed  (2's comp)"  n_bits=39  bin_pt=28  quantization=Truncate  overflow=Wrap  use_behavioral_HDL=off  hw_selection=Fabric  pipelined=off  dbl_ovrd=off  block_type=addsub
  AddSub4 : xbsIndex_r4/AddSub  mode=Addition  use_carryin=off  use_carryout=off  en=off  latency=0  precision=User Defined  arith_type="Signed  (2's comp)"  n_bits=38  bin_pt=28  quantization=Truncate  overflow=Wrap  use_behavioral_HDL=off  hw_selection=Fabric  pipelined=off  dbl_ovrd=off  block_type=addsub
  CMult : xbsIndex_r4/CMult  const=K1  gui_display_data_type=Fixed-point  const_n_bits=15  const_bin_pt=14  float_type=Single  exp_bits=8  fraction_bits=24  en=off  latency=0  precision=Full  arith_type="Signed  (2's comp)"  n_bits=18  bin_pt=14  quantization=Truncate  overflow=Wrap  use_behavioral_HDL=off  mem_type=Distributed RAM  pipeline=off  dbl_ovrd=off  block_type=cmult
  CMult1 : xbsIndex_r4/CMult  const=K2  gui_display_data_type=Fixed-point  const_n_bits=18  const_bin_pt=14  float_type=Single  exp_bits=8  fraction_bits=24  en=off  latency=0  precision=Full  arith_type="Signed  (2's comp)"  n_bits=18  bin_pt=14  quantization=Truncate  overflow=Wrap  use_behavioral_HDL=off  mem_type=Distributed RAM  pipeline=off  dbl_ovrd=off  block_type=cmult
  Constant : xbsIndex_r4/Constant  const=0  gui_display_data_type=Fixed-point  arith_type=Signed (2's comp)  n_bits=16  bin_pt=14  preci_type=Single  exp_width=8  frac_width=24  explicit_period=on  period=1/(Rsymbol*OSR)  equ=P=C  opselect=C  inp2=PCIN>>17  opr=+  inp1=P  carry=CIN  dbl_ovrd=off  block_type=constant
  Delay : xbsIndex_r4/Delay  rst=off  infoeditControl=Selection of Reset will increase slice count due to use of real FFs and instead of SRLs  en=off  latency=1  reg_retiming=off  dbl_ovrd=off  block_type=delay
  Mux : xbsIndex_r4/Mux  inputs=2  en=off  latency=0  precision=Full  arith_type="Signed  (2's comp)"  n_bits=18  bin_pt=14  quantization=Truncate  overflow=Wrap  dbl_ovrd=off  block_type=mux
  Register1 : xbsIndex_r4/Register  init=0  rst=on  en=on  dbl_ovrd=off  block_type=register
  Error_Filt : Outport
  En_out : Outport  Port=2
  wires:
  Register1/1 -> AddSub4/2
  CMult1/1 -> AddSub4/1
  CMult/1 -> AddSub3/1
  Mux/1 -> Register1/1
  Signal/1 -> CMult1/1, CMult/1
  AddSub4/1 -> Mux/3, AddSub3/2
  En_in/1 -> Register1/3, Delay/1, Mux/1
  Constant/1 -> Mux/2
  AddSub3/1 -> Error_Filt/1
  Delay/1 -> En_out/1
  reset/1 -> Register1/2

== system axi_qpsk_rx_tsync/Carrier Synch/NCO ==
  Step Size : Inport
  En_in : Inport  Port=2
  AddSub4 : xbsIndex_r4/AddSub  mode=Addition  use_carryin=off  use_carryout=off  en=off  latency=0  precision=User Defined  arith_type="Signed  (2's comp)"  n_bits=n+b  bin_pt=b  quantization=Truncate  overflow=Wrap  use_behavioral_HDL=off  hw_selection=Fabric  pipelined=off  dbl_ovrd=off  block_type=addsub
  CMult1 : xbsIndex_r4/CMult  const=(2^n)/(2*pi)  gui_display_data_type=Fixed-point  const_n_bits=k_n+b  const_bin_pt=b  float_type=Single  exp_bits=8  fraction_bits=24  en=off  latency=0  precision=User Defined  arith_type="Signed  (2's comp)"  n_bits=n+b  bin_pt=b  quantization=Truncate  overflow=Wrap  use_behavioral_HDL=off  mem_type=Distributed RAM  pipeline=off  dbl_ovrd=off  block_type=cmult
  Constant : xbsIndex_r4/Constant  const=0  gui_display_data_type=Fixed-point  arith_type=Signed (2's comp)  n_bits=16  bin_pt=14  preci_type=Single  exp_width=8  frac_width=24  explicit_period=on  period=1/(Rsymbol*OSR)  equ=P=C  opselect=C  inp2=PCIN>>17  opr=+  inp1=P  carry=CIN  dbl_ovrd=off  block_type=constant
  Convert1 : xbsIndex_r4/Convert  gui_display_data_type=Fixed-point  arith_type=Unsigned  n_bits=n  bin_pt=0  float_type=Single  exp_bits=8  fraction_bits=24  quantization=Truncate  overflow=Wrap  en=off  latency=0  pipeline=off  dbl_ovrd=off  block_type=convert
  Cos ROM : xbsIndex_r4/ROM  depth=2^n  initVector=cos(pi*(0:((2^n)-1))/(2^(n-1)))  distributed_mem=Block RAM  rst=off  init_reg=0  en=off  latency=1  gui_display_data_type=Fixed-point  arith_type="Signed  (2's comp)"  n_bits=16  bin_pt=14  preci_type=Single  exp_width=8  frac_width=24  optimize=Area  use_rpm=on  dbl_ovrd=off  block_type=sprom
  Delay : xbsIndex_r4/Delay  rst=off  infoeditControl=Selection of Reset will increase slice count due to use of real FFs and instead of SRLs  en=off  latency=1  reg_retiming=off  dbl_ovrd=off  block_type=delay
  Mux : xbsIndex_r4/Mux  inputs=2  en=off  latency=0  precision=Full  arith_type="Signed  (2's comp)"  n_bits=18  bin_pt=14  quantization=Truncate  overflow=Wrap  dbl_ovrd=off  block_type=mux
  Neg Sin ROM : xbsIndex_r4/ROM  depth=2^n  initVector=-sin(pi*(0:((2^n)-1))/(2^(n-1)))  distributed_mem=Block RAM  rst=off  init_reg=0  en=off  latency=1  gui_display_data_type=Fixed-point  arith_type="Signed  (2's comp)"  n_bits=16  bin_pt=14  preci_type=Single  exp_width=8  frac_width=24  optimize=Area  use_rpm=on  dbl_ovrd=off  block_type=sprom
  Register1 : xbsIndex_r4/Register  init=0  rst=off  en=on  dbl_ovrd=off  block_type=register
  Cos : Outport
  Neg Sin : Outport  Port=2
  En_out : Outport  Port=3
  wires:
  Delay/1 -> En_out/1
  Cos ROM/1 -> Cos/1
  Constant/1 -> Mux/2
  En_in/1 -> Delay/1, Mux/1, Register1/2
  Step Size/1 -> CMult1/1
  Mux/1 -> Register1/1
  CMult1/1 -> AddSub4/1
  Register1/1 -> AddSub4/2
  Neg Sin ROM/1 -> Neg Sin/1
  AddSub4/1 -> Convert1/1, Mux/3
  Convert1/1 -> Neg Sin ROM/1, Cos ROM/1

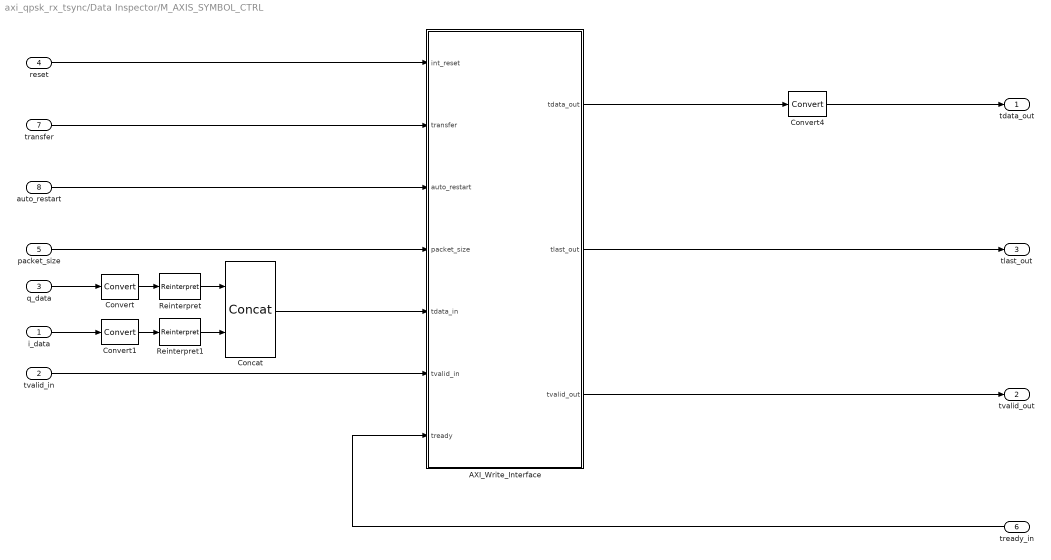
== system axi_qpsk_rx_tsync/Data Inspector/M_AXIS_SYMBOL_CTRL ==
  i_data : Inport
  tvalid_in : Inport  Port=2
  q_data : Inport  Port=3
  reset : Inport  Port=4
  packet_size : Inport  Port=5
  tready_in : Inport  Port=6
  transfer : Inport  Port=7
  auto_restart : Inport  Port=8
  AXI_Write_Interface : Subsystem
  Concat : xbsIndex_r4/Concat  num_inputs=2  dbl_ovrd=off  block_type=concat
  Convert : xbsIndex_r4/Convert  gui_display_data_type=Fixed-point  arith_type="Signed  (2's comp)"  n_bits=16  bin_pt=14  float_type=Single  exp_bits=8  fraction_bits=24  quantization=Truncate  overflow=Wrap  en=off  latency=0  pipeline=off  dbl_ovrd=off  block_type=convert
  Convert1 : xbsIndex_r4/Convert  gui_display_data_type=Fixed-point  arith_type="Signed  (2's comp)"  n_bits=16  bin_pt=14  float_type=Single  exp_bits=8  fraction_bits=24  quantization=Truncate  overflow=Wrap  en=off  latency=0  pipeline=off  dbl_ovrd=off  block_type=convert
  Convert4 : xbsIndex_r4/Convert  gui_display_data_type=Fixed-point  arith_type=Unsigned  n_bits=32  bin_pt=0  float_type=Single  exp_bits=8  fraction_bits=24  quantization=Truncate  overflow=Wrap  en=off  latency=0  pipeline=off  dbl_ovrd=off  block_type=convert
  Reinterpret : xbsIndex_r4/Reinterpret  force_arith_type=on  arith_type=Unsigned  force_bin_pt=on  bin_pt=0  block_type=reinterpret
  Reinterpret1 : xbsIndex_r4/Reinterpret  force_arith_type=on  arith_type=Unsigned  force_bin_pt=on  bin_pt=0  block_type=reinterpret
  tdata_out : Outport
  tvalid_out : Outport  Port=2
  tlast_out : Outport  Port=3
  wires:
  Convert4/1 -> tdata_out/1
  AXI_Write_Interface/1(tdata_out) -> Convert4/1
  AXI_Write_Interface/3(tvalid_out) -> tvalid_out/1
  AXI_Write_Interface/2(tlast_out) -> tlast_out/1
  tready_in/1 -> AXI_Write_Interface/7(tready)
  auto_restart/1 -> AXI_Write_Interface/3(auto_restart)
  transfer/1 -> AXI_Write_Interface/2(transfer)
  Concat/1 -> AXI_Write_Interface/5(tdata_in)
  reset/1 -> AXI_Write_Interface/1(int_reset)
  tvalid_in/1 -> AXI_Write_Interface/6(tvalid_in)
  packet_size/1 -> AXI_Write_Interface/4(packet_size)
  Reinterpret/1 -> Concat/1
  Reinterpret1/1 -> Concat/2
  i_data/1 -> Convert1/1
  q_data/1 -> Convert/1
  Convert/1 -> Reinterpret/1
  Convert1/1 -> Reinterpret1/1

== system axi_qpsk_rx_tsync/Timing Synch/Loop Filter ==
  Signal : Inport
  En : Inport  Port=2
  reset : Inport  Port=3
  AddSub3 : xbsIndex_r4/AddSub  mode=Addition  use_carryin=off  use_carryout=off  en=off  latency=0  precision=User Defined  arith_type="Signed  (2's comp)"  n_bits=39  bin_pt=28  quantization=Truncate  overflow=Wrap  use_behavioral_HDL=off  hw_selection=Fabric  pipelined=off  dbl_ovrd=off  block_type=addsub
  AddSub4 : xbsIndex_r4/AddSub  mode=Addition  use_carryin=off  use_carryout=off  en=off  latency=0  precision=User Defined  arith_type="Signed  (2's comp)"  n_bits=38  bin_pt=28  quantization=Truncate  overflow=Wrap  use_behavioral_HDL=off  hw_selection=Fabric  pipelined=off  dbl_ovrd=off  block_type=addsub
  CMult : xbsIndex_r4/CMult  const=Ka  gui_display_data_type=Fixed-point  const_n_bits=15  const_bin_pt=14  float_type=Single  exp_bits=8  fraction_bits=24  en=off  latency=0  precision=Full  arith_type="Signed  (2's comp)"  n_bits=18  bin_pt=14  quantization=Truncate  overflow=Wrap  use_behavioral_HDL=off  mem_type=Distributed RAM  pipeline=off  dbl_ovrd=off  block_type=cmult
  CMult1 : xbsIndex_r4/CMult  const=Kb  gui_display_data_type=Fixed-point  const_n_bits=18  const_bin_pt=14  float_type=Single  exp_bits=8  fraction_bits=24  en=off  latency=0  precision=Full  arith_type="Signed  (2's comp)"  n_bits=18  bin_pt=14  quantization=Truncate  overflow=Wrap  use_behavioral_HDL=off  mem_type=Distributed RAM  pipeline=off  dbl_ovrd=off  block_type=cmult
  Constant : xbsIndex_r4/Constant  const=0  gui_display_data_type=Fixed-point  arith_type=Signed (2's comp)  n_bits=16  bin_pt=14  preci_type=Single  exp_width=8  frac_width=24  explicit_period=on  period=1/(Rsymbol*OSR)  equ=P=C  opselect=C  inp2=PCIN>>17  opr=+  inp1=P  carry=CIN  dbl_ovrd=off  block_type=constant
  Mux : xbsIndex_r4/Mux  inputs=2  en=off  latency=0  precision=Full  arith_type="Signed  (2's comp)"  n_bits=18  bin_pt=14  quantization=Truncate  overflow=Wrap  dbl_ovrd=off  block_type=mux
  Register1 : xbsIndex_r4/Register  init=0  rst=on  en=on  dbl_ovrd=off  block_type=register
  Error_Filt : Outport
  wires:
  Register1/1 -> AddSub4/2
  CMult1/1 -> AddSub4/1
  CMult/1 -> AddSub3/1
  Mux/1 -> Register1/1
  Signal/1 -> CMult1/1, CMult/1
  AddSub4/1 -> Mux/3, AddSub3/2
  En/1 -> Register1/3, Mux/1
  Constant/1 -> Mux/2
  AddSub3/1 -> Error_Filt/1
  reset/1 -> Register1/2

== system axi_qpsk_rx_tsync/Timing Synch/NCC ==
  note: OSR might not be a power of 2
      | (so simply detecting wrap is not sufficient).
      |
      | Section to left is equivalent to modulo (OSR).
  Error_Filt : Inport
  En : Inport  Port=2
  AddSub1 : xbsIndex_r4/AddSub  mode=Subtraction  use_carryin=off  use_carryout=off  en=off  latency=0  precision=User Defined  arith_type=Unsigned  n_bits=n+b  bin_pt=b  quantization=Truncate  overflow=Wrap  use_behavioral_HDL=off  hw_selection=Fabric  pipelined=off  dbl_ovrd=off  block_type=addsub
  AddSub5 : xbsIndex_r4/AddSub  mode=Addition  use_carryin=off  use_carryout=off  en=off  latency=0  precision=User Defined  arith_type=Unsigned  n_bits=n+b+1  bin_pt=b  quantization=Truncate  overflow=Wrap  use_behavioral_HDL=off  hw_selection=Fabric  pipelined=off  dbl_ovrd=off  block_type=addsub
  AddSub6 : xbsIndex_r4/AddSub  mode=Addition  use_carryin=off  use_carryout=off  en=off  latency=0  precision=User Defined  arith_type=Unsigned  n_bits=2+b  bin_pt=b  quantization=Truncate  overflow=Wrap  use_behavioral_HDL=off  hw_selection=Fabric  pipelined=off  dbl_ovrd=off  block_type=addsub
  Constant1 : xbsIndex_r4/Constant  const=1.0  gui_display_data_type=Fixed-point  arith_type=Unsigned  n_bits=b+2  bin_pt=b  preci_type=Single  exp_width=8  frac_width=24  explicit_period=on  period=1/(Rsymbol*OSR)  equ=P=C  opselect=C  inp2=PCIN>>17  opr=+  inp1=P  carry=CIN  dbl_ovrd=off  block_type=constant
  Constant2 : xbsIndex_r4/Constant  const=OSR  gui_display_data_type=Fixed-point  arith_type=Unsigned  n_bits=n+b+1  bin_pt=b  preci_type=Single  exp_width=8  frac_width=24  explicit_period=on  period=1/(Rsymbol*OSR)  equ=P=C  opselect=C  inp2=PCIN>>17  opr=+  inp1=P  carry=CIN  dbl_ovrd=off  block_type=constant
  Mux : xbsIndex_r4/Mux  inputs=2  en=off  latency=0  precision=User Defined  arith_type=Unsigned  n_bits=n+b  bin_pt=b  quantization=Truncate  overflow=Wrap  dbl_ovrd=off  block_type=mux
  Register : xbsIndex_r4/Register  init=2  rst=off  en=on  dbl_ovrd=off  block_type=register
  Relational : xbsIndex_r4/Relational  mode=a>b  op_type=Bool  en=off  latency=0  dbl_ovrd=off  block_type=relational
  Relational1 : xbsIndex_r4/Relational  mode=a>b  op_type=Bool  en=off  latency=0  dbl_ovrd=off  block_type=relational
  Strobe : Outport
  Adj_Step : Outport  Port=2
  wires:
  Register/1 -> Mux/2, Relational1/1, AddSub1/1, Relational/1
  Relational/1 -> Strobe/1
  Constant1/1 -> AddSub6/2
  Error_Filt/1 -> AddSub6/1
  AddSub6/1 -> Adj_Step/1, AddSub5/2
  AddSub5/1 -> Register/1, Relational/2
  Mux/1 -> AddSub5/1
  AddSub1/1 -> Mux/3
  Relational1/1 -> Mux/1
  Constant2/1 -> AddSub1/2, Relational1/2
  En/1 -> Register/2

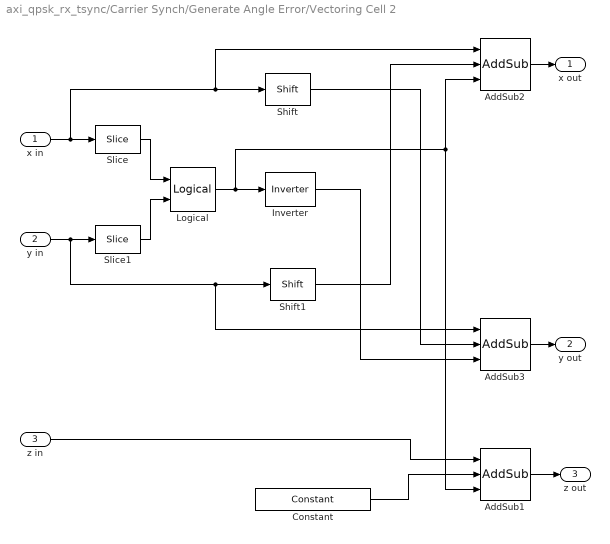
== system axi_qpsk_rx_tsync/Carrier Synch/Generate Angle Error/Vectoring Cell 2 ==
  x in : Inport
  y in : Inport  Port=2
  z in : Inport  Port=3
  AddSub1 : xbsIndex_r4/AddSub  mode=Addition or Subtraction  use_carryin=off  use_carryout=off  en=off  latency=0  precision=User Defined  arith_type="Signed  (2's comp)"  n_bits=20  bin_pt=18  quantization=Truncate  overflow=Wrap  use_behavioral_HDL=on  hw_selection=Fabric  pipelined=off  use_rpm=on  dbl_ovrd=off  block_type=addsub
      settings: xl_area=[0, 0, 0, 0, 0, 0, 0]  block_version=VER_STRING_GOES_HERE
  AddSub2 : xbsIndex_r4/AddSub  mode=Addition or Subtraction  use_carryin=off  use_carryout=off  en=off  latency=0  precision=User Defined  arith_type="Signed  (2's comp)"  n_bits=15  bin_pt=12  quantization=Truncate  overflow=Wrap  use_behavioral_HDL=on  hw_selection=Fabric  pipelined=off  use_rpm=on  dbl_ovrd=off  block_type=addsub
      settings: xl_area=[0, 0, 0, 0, 0, 0, 0]  block_version=VER_STRING_GOES_HERE
  AddSub3 : xbsIndex_r4/AddSub  mode=Addition or Subtraction  use_carryin=off  use_carryout=off  en=off  latency=0  precision=User Defined  arith_type="Signed  (2's comp)"  n_bits=15  bin_pt=12  quantization=Truncate  overflow=Wrap  use_behavioral_HDL=on  hw_selection=Fabric  pipelined=off  use_rpm=on  dbl_ovrd=off  block_type=addsub
      settings: xl_area=[0, 0, 0, 0, 0, 0, 0]  block_version=VER_STRING_GOES_HERE
  Constant : xbsIndex_r4/Constant  const=atan(2^-i)  gui_display_data_type=Fixed-point  arith_type=Signed (2's comp)  n_bits=20  bin_pt=18  preci_type=Single  exp_width=8  frac_width=24  explicit_period=off  period=1  equ=P=C  opselect=C  inp2=PCIN>>17  opr=+  inp1=P  carry=CIN  dbl_ovrd=off  block_type=constant
      settings: block_version=10.1.2
  Inverter : xbsIndex_r4/Inverter  en=off  latency=0  dbl_ovrd=off  block_type=inv
      settings: xl_area=[0, 0, 0, 0, 0, 0, 0]  block_version=VER_STRING_GOES_HERE
  Logical : xbsIndex_r4/Logical  logical_function=XOR  inputs=2  en=off  latency=0  precision=Full  arith_type=Unsigned  n_bits=1  bin_pt=0  align_bp=on  dbl_ovrd=off  block_type=logical
      settings: xl_area=[0, 0, 0, 0, 0, 0, 0]  block_version=VER_STRING_GOES_HERE
  Shift : xbsIndex_r4/Shift  shift_dir=Right  shift_bits=i  en=off  latency=0  precision=User Defined  arith_type="Signed  (2's comp)"  n_bits=15  bin_pt=12  quantization=Truncate  overflow=Wrap  dbl_ovrd=off  block_type=shift
      settings: xl_area=[0, 0, 0, 0, 0, 0, 0]  block_version=VER_STRING_GOES_HERE
  Shift1 : xbsIndex_r4/Shift  shift_dir=Right  shift_bits=i  en=off  latency=0  precision=User Defined  arith_type="Signed  (2's comp)"  n_bits=15  bin_pt=12  quantization=Truncate  overflow=Wrap  dbl_ovrd=off  block_type=shift
      settings: xl_area=[0, 0, 0, 0, 0, 0, 0]  block_version=VER_STRING_GOES_HERE
  Slice : xbsIndex_r4/Slice  nbits=1  boolean_output=on  mode=Upper Bit Location + Width  bit1=0  base1=MSB of Input  bit0=0  base0=LSB of Input  dbl_ovrd=off  block_type=slice
      settings: infoedit="Extracts a given range of bits from each input sample and presents it at the output.  The output type is ordinarily unsigned with binary point at zero, but can be Boolean when the slice is one bit wide.<P><P>Hardware notes: In hardware this block costs nothing."  block_version=VER_STRING_GOES_HERE
  Slice1 : xbsIndex_r4/Slice  nbits=1  boolean_output=on  mode=Upper Bit Location + Width  bit1=0  base1=MSB of Input  bit0=0  base0=LSB of Input  dbl_ovrd=off  block_type=slice
      settings: infoedit="Extracts a given range of bits from each input sample and presents it at the output.  The output type is ordinarily unsigned with binary point at zero, but can be Boolean when the slice is one bit wide.<P><P>Hardware notes: In hardware this block costs nothing."  block_version=VER_STRING_GOES_HERE
  x out : Outport
  y out : Outport  Port=2
  z out : Outport  Port=3
  wires:
  x in/1 -> AddSub2/1, Shift/1, Slice/1
  y in/1 -> AddSub3/1, Shift1/1, Slice1/1
  Slice/1 -> Logical/1
  Slice1/1 -> Logical/2
  Logical/1 -> Inverter/1, AddSub2/3, AddSub1/3
  Shift1/1 -> AddSub2/2
  Shift/1 -> AddSub3/2
  Inverter/1 -> AddSub3/3
  AddSub2/1 -> x out/1
  AddSub3/1 -> y out/1
  z in/1 -> AddSub1/1
  Constant/1 -> AddSub1/2
  AddSub1/1 -> z out/1
